simulink model "section_4_4"  (R2021b)
settings: Solver=VariableStepAuto  StartTime=0.0  StopTime=10.0  RelTol=1e-3
libraries: cstblocks x2
settings Model: Creator=varunsampat  LastModifiedBy=varunsampat

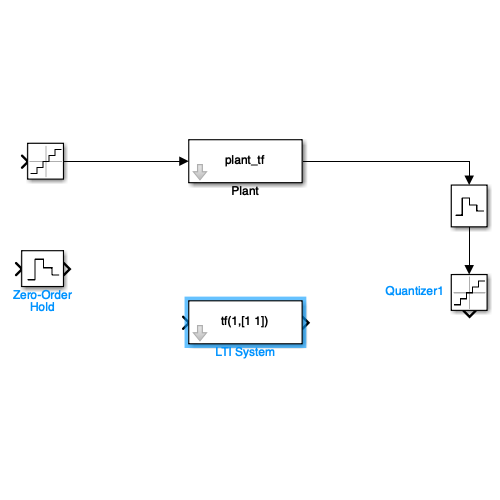
[thumbnail: Simulink's stored preview of the top-level diagram]
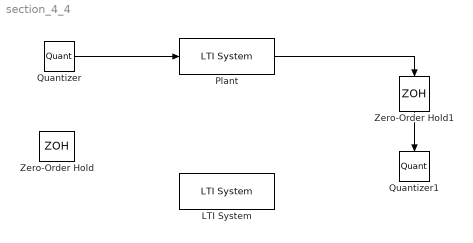
== system section_4_4 ==
  LTI System : cstblocks/LTI System  sys=tf(1,[1 1])  IC=[]
  Plant : cstblocks/LTI System  sys=plant_tf  IC=[]
  Quantizer : Quantizer
  Quantizer1 : Quantizer
  Zero-Order Hold : ZeroOrderHold  SampleTime=-1
  Zero-Order Hold1 : ZeroOrderHold  SampleTime=-1
  wires:
  Quantizer/1 -> Plant/1
  Plant/1 -> Zero-Order Hold1/1
  Zero-Order Hold1/1 -> Quantizer1/1
